simulink library "Powertrain_Library_GenAI"  (R2024a)
settings: Solver=VariableStepAuto  StartTime=0.0  StopTime=10.0  RelTol=1e-3
undefined symbols (not defined in the file or in its folder): DriveCycle
libraries: simulink x8, slpidlib x1
(part 1 of 2)
settings Model: Creator=LENOVO THINKPAD  LastModifiedBy=malikr2
settings RTWCC: GPUComputeCapability=3.5

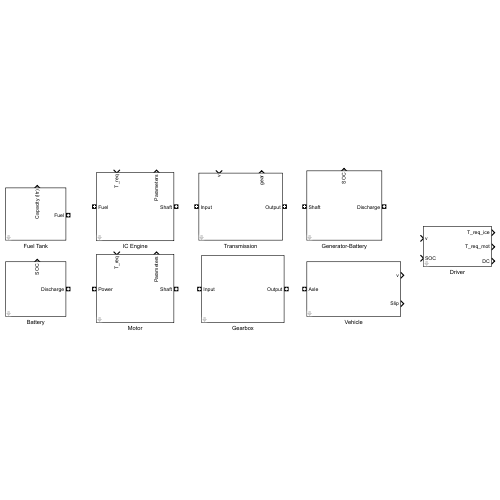
[thumbnail: Simulink's stored preview of the top-level diagram]
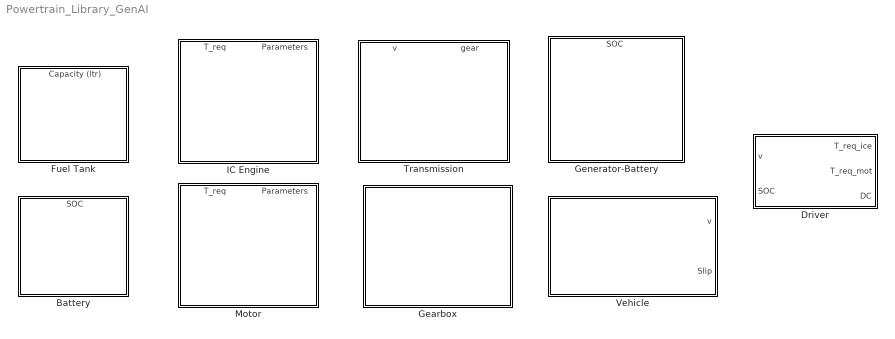
== system Powertrain_Library_GenAI ==
  Battery : Subsystem  mask{V_bat_nom=228, R_bat=0.1037, mAh_bat_rated=87500, SOC_bat_0=1, min_SOC=0.2, attribute_vector={'STORE', 'BAT', '1', {'ELEC'}, {'OUT'}}, cost=4000, base_emissions=8000}
      mask prompts: V_bat_nom "Battery Nominal Voltage (V)"; R_bat "Battery Internal Resistance (Ohm)"; mAh_bat_rated "Battery Capacity (mAh)"; SOC_bat_0 "Initial SOC"; min_SOC "Minimum Operable SOC"; cost "Cost (Euros)"; base_emissions "Production Emissions (kg of CO2)"
      settings: PortSchema="{\"entries\":[{\"content\":{\"sides\":[{\"content\":{},\"type\":\"ConnectorPlacement.EquallySpacedRectSide\",\"uuid\":\"791ecc86-3bcc-4c6a-a153-95c10547b091\"},{\"content\":{\"connectorIds\":[\"RConn1\"],\"side\":\"RIGHT\"},\"type\":\"ConnectorPlacement.EquallySpacedRectSide\",\"uuid\":\"8e54d6b5-5ca6-4d71-8ac9-0532fb867ed6\"},{\"content\":{\"connectorIds\":[\"Out1\"],\"side\":\"TOP\"},\"type\":\"ConnectorPlacement.EquallySpacedRectSide\",\"uuid\":\"933f38fd-4181-4d8b-8acd-50ce6fa4b91a\"}]},\"type\":\"ConnectorPlacement.EquallySpacedConnector\",\"uuid\":\"308b2aba-12b6-4e08-8192-d5b89fa1859a\"}],\"packageUris\":[\"http://schema.mathworks.com/mf0/Connector/R2020b\"],\"version\":\"1.0\"}"
      mask DialogControl Container3 Prompt: Economic Parameters
  Driver : Subsystem  mask{K_p=0, K_i=0, K_d=0, drive_cycle=DriveCycle, ITAE=0, attribute_vector={'CONTROLLER', 'DRV', '0', {}, ''}, series_hybrid_mode=0, charging_torque=50, charging_time=60, min_charge_SOC=0.5}
      mask prompts: K_p "Proportional Gain"; K_i "Integral Gain"; K_d "Derivative Gain"; drive_cycle "Drive Cycle"; series_hybrid_mode "Series Hybrid Mode"; charging_torque "Charging Torque (Nm)"; charging_time "Charging time (seconds)"; min_charge_SOC "Min. SOC to start charging"
      mask DialogControl Container3 Prompt: Hybrid Control
  Fuel Tank : Subsystem  mask{Parameter1=0, attribute_vector={'STORE', 'FT', '1', {'CHEM'}, {'OUT'}}, fuel_energy_density=46, fuel_density=750, fuel_capacity=4, cost=300, base_emissions=200}
      mask prompts: fuel_energy_density "Fuel Energy Density (MJ/kg)"; fuel_density "Fuel Density (kg/m^3)"; fuel_capacity "Tank Capacity (litres)"; cost "Cost (Euros)"; base_emissions "Production Emissions (kg of CO2)"
      settings: PortSchema="{\"entries\":[{\"content\":{\"sides\":[{\"content\":{},\"type\":\"ConnectorPlacement.EquallySpacedRectSide\",\"uuid\":\"791ecc86-3bcc-4c6a-a153-95c10547b091\"},{\"content\":{\"connectorIds\":[\"RConn1\"],\"side\":\"RIGHT\"},\"type\":\"ConnectorPlacement.EquallySpacedRectSide\",\"uuid\":\"8e54d6b5-5ca6-4d71-8ac9-0532fb867ed6\"},{\"content\":{\"connectorIds\":[\"Out1\"],\"side\":\"TOP\"},\"type\":\"ConnectorPlacement.EquallySpacedRectSide\",\"uuid\":\"933f38fd-4181-4d8b-8acd-50ce6fa4b91a\"}]},\"type\":\"ConnectorPlacement.EquallySpacedConnector\",\"uuid\":\"308b2aba-12b6-4e08-8192-d5b89fa1859a\"}],\"packageUris\":[\"http://schema.mathworks.com/mf0/Connector/R2020b\"],\"version\":\"1.0\"}"
      mask DialogControl Container3 Prompt: Economic Parameters
  Gearbox : Subsystem  mask{G=9, eff_gb=0.96, attribute_vector={'TRANSMIT', 'GB', '2', {'MECH', 'MECH'}, {'IN','OUT'}}, cost=1200, base_emissions=1000}
      mask prompts: G "Gear Ratio"; eff_gb "Gearbox Efficiency"; cost "Cost (Euros)"; base_emissions "Production Emissions (kg of CO2)"
      mask DialogControl Container3 Prompt: Economic Parameters
  Generator-Battery : Subsystem  mask{eff_gen=0.85, generator_rpm=6000, V_bat_nom=228, R_bat=0.1037, mAh_bat_rated=87500, SOC_bat_0=0.6, min_SOC=0.2, attribute_vector={'GENERATOR', 'GEN', '2', {'MECH','ELEC'}, {'IN','OUT'}}, cost=7500, base_emissions=10000}
      mask prompts: eff_gen "Generator Efficiency"; generator_rpm "Generator Working Speed (RPM)"; V_bat_nom "Battery Nominal Voltage (V)"; R_bat "Battery Internal Resistance (Ohm)"; mAh_bat_rated "Battery Capacity (mAh)"; SOC_bat_0 "Initial SOC"; min_SOC "Minimum Operable SOC"; cost "Cost (Euros)"; base_emissions "Production Emissions (kg of CO2)"
      settings: PortSchema="{\"entries\":[{\"content\":{\"sides\":[{\"content\":{\"connectorIds\":[\"LConn1\"]},\"type\":\"ConnectorPlacement.EquallySpacedRectSide\",\"uuid\":\"a8b73504-e9cb-44b1-bc91-1a2623164e75\"},{\"content\":{\"connectorIds\":[\"RConn1\"],\"side\":\"RIGHT\"},\"type\":\"ConnectorPlacement.EquallySpacedRectSide\",\"uuid\":\"a3351110-409d-4b78-bb75-8efa6d683458\"},{\"content\":{\"connectorIds\":[\"Out1\"],\"side\":\"TOP\"},\"type\":\"ConnectorPlacement.EquallySpacedRectSide\",\"uuid\":\"2c783bb7-545b-4095-8c4d-b76f612407dc\"}]},\"type\":\"ConnectorPlacement.EquallySpacedConnector\",\"uuid\":\"3e5aa339-5af4-4070-a704-22faf7e6b2c2\"}],\"packageUris\":[\"http://schema.mathworks.com/mf0/Connector/R2020b\"],\"version\":\"1.0\"}"
      mask DialogControl Container4 Prompt: Generator Parameters
      mask DialogControl ParameterGroupVar Prompt: Battery Parameters
      mask DialogControl Container3 Prompt: Economic Parameters
  IC Engine : Subsystem  mask{torque_modelling=Normalized 3rd-order polynomial approximation, efficiency_modelling=Variable Efficiency, attribute_vector={'ACTUATOR', 'ICE', '2', {'CHEM','MECH'}, {'IN','OUT'}}, P_p=125000, T_p=228, w_P=6000, w_T=4500, w_ice_max=7000, w_ice_stall=1000, T_ice_data=[180, 192, 207, 215, 220, 225, 228, 226, 220, 210, 200, 182, 162], w_ice_data=[1000, 1500, 2000, 2500, 3000, 3500, 4000, 4500, 5000, 5500, 6000, 6500, 7000], eff_ice_avg=0.25, eff_ice_data=[0.0900 0.0900 0.0900 0.0900 0.0900 0.0900 0.0850 0.0800 0.0750 0.0700 0.0500;         0.1700 0.1700 0.1700 0.1700 0.1600 0.1500 0.1400 0.1300 0.1200 0.1100 0.0900;         0.2100 0.2100 0.2100 0.2100 0.2100 0.2050 0.2000 0.1800 0.1650 0.1500 0.1300;         0.2500 0.2500 0.2500 0.2500 0.2400 0.2350 0.2200 0.2050 0.1900 0.1700 0.1500;         0.2650 0.2700 0.2700 0.2700 0.2650 0.2500 0.2450 0.2350 0.2150 0.1950 0.1700;         0.2800 0.2800 0.2800 0.2800 0.2800 0.2700 0.2650 0.2500 0.2300 0.2100 0.1900;         0.3000 0.3000 0.3000 0.3000 0.3000 0.3000 0.2900 0.2700 0.2500 0.2150 0.1900;         0.3200 0.3300 0.3300 0.3300 0.3300 0.3300 0.3100 0.2750 0.2400 0.2050 0.1800;         0.2900 0.3100 0.3400 0.3400 0.3300 0.3000 0.2700 0.2500 0.2300 0.1900 0.1700;         0.2500 0.2800 0.3150 0.3150 0.2900 0.2700 0.2500 0.2300 0.2200 0.1800 0.1600;         0.2500 0.2800 0.3150 0.3150 0.2900 0.2700 0.2500 0.2300 0.2200 0.1800 0.1600], T_ice_norm_data=[0; 25; 50; 75; 100; 125; 150; 175; 200; 225; 228]/228, w_ice_norm_data=[1000 1600 2200 2800 3400 4000 4600 5200 5800 6300 7000]/7000, cost=2500, base_emissions=3000}
      mask prompts: torque_modelling "Model Parameterization"; efficiency_modelling "Efficiency Modelling"; P_p "Max. Power (W)"; T_p "Max. Torque (Nm)"; w_P "Speed @ Max. Power (rpm)"; w_T "Speed @ Max. Torque (rpm)"; w_ice_max "Max. Speed (rpm)"; w_ice_stall "Stall Speed (rpm)"; T_ice_data "Torque values (Nm)"; w_ice_data "Speed breakpoints (rpm)"; eff_ice_avg "Average Engine Efficiency"; eff_ice_data "Engine Efficiency map data"; T_ice_norm_data "Torque breakpoints (normalized w.r.t max. torque)"; w_ice_norm_data "Speed breakpoints (normalized w.r.t max. speed)"; cost "Cost (Euros)"; base_emissions "Production Emissions (kg of CO2)"
      settings: PortSchema="{\"entries\":[{\"content\":{\"sides\":[{\"content\":{\"connectorIds\":[\"LConn1\"]},\"type\":\"ConnectorPlacement.EquallySpacedRectSide\",\"uuid\":\"10ac0862-84c0-40da-a453-235e59b4628d\"},{\"content\":{\"connectorIds\":[\"RConn1\"],\"side\":\"RIGHT\"},\"type\":\"ConnectorPlacement.EquallySpacedRectSide\",\"uuid\":\"cd810463-95cc-48e1-84e4-d50e07225fce\"},{\"content\":{\"connectorIds\":[\"In1\",\"Out1\"],\"side\":\"TOP\"},\"type\":\"ConnectorPlacement.EquallySpacedRectSide\",\"uuid\":\"990bc9f6-9b76-43af-8727-286cb1281cc3\"}]},\"type\":\"ConnectorPlacement.EquallySpacedConnector\",\"uuid\":\"ec51f7b2-97ac-4e7c-b90f-37b44cc14701\"}],\"packageUris\":[\"http://schema.mathworks.com/mf0/Connector/R2020b\"],\"version\":\"1.0\"}"
      mask TypeOptions torque_modelling: ICE_Torque_Limits/torque_modelling
      mask TypeOptions efficiency_modelling: ICE_Efficiency/efficiency_modelling
      mask TypeOptions P_p: ICE_Torque_Limits/P_p
      mask TypeOptions T_p: ICE_Torque_Limits/T_p
      mask TypeOptions w_P: ICE_Torque_Limits/w_P
      mask TypeOptions w_T: ICE_Torque_Limits/w_T
      mask TypeOptions w_ice_max: ICE_Torque_Limits/w_ice_max
      mask TypeOptions w_ice_stall: ICE_Torque_Limits/w_ice_stall
      mask TypeOptions T_ice_data: ICE_Torque_Limits/T_ice_data
      mask TypeOptions w_ice_data: ICE_Torque_Limits/w_ice_data
      mask TypeOptions eff_ice_avg: ICE_Efficiency/eff_ice_avg
      mask TypeOptions eff_ice_data: ICE_Efficiency/eff_ice_data
      mask TypeOptions T_ice_norm_data: ICE_Efficiency/T_ice_norm_data
      mask TypeOptions w_ice_norm_data: ICE_Efficiency/w_ice_norm_data
      mask DialogControl Container3 Prompt: Polynomial Approximation Parameters
      mask DialogControl Container4 Prompt: Torque Curve Data
      mask DialogControl Control2 Prompt: Torque Curve
      mask DialogControl Container6 Prompt: Constant Efficiency Modelling
      mask DialogControl Container5 Prompt: Efficiency Map Modelling
      mask DialogControl Container7 Prompt: Economic Parameters
      mask DialogControl Control3 Prompt: Efficiency Map
  Motor : Subsystem  mask{attribute_vector={'ACTUATOR', 'MOT', '2', {'ELEC','MECH'}, {'IN','OUT'}}, mot_efficiency_modelling=Constant Efficiency, T_mot_max=265, P_mot_max=140000, w_mot_max=20000, eff_mot_avg=0.85, eff_mot_data=[0.5833    0.6122    0.7211    0.7696    0.7951    0.8158    0.8293    0.8392    0.8475    0.8519    0.8536    0.8549    0.8563    0.8593    0.8607    0.8605    0.8610    0.8604    0.8590    0.8578    0.8583    0.8582    0.8571    0.8549    0.8535    0.8511    0.8486    0.8479    0.8478    0.8475    0.8431    0.8384    0.8350;     0.5833    0.6122    0.7211    0.7696    0.7951    0.8158    0.8293    0.8392    0.8475    0.8519    0.8536    0.8549    0.8563    0.8593    0.8607    0.8605    0.8610    0.8604    0.8590    0.8578    0.8583    0.8582    0.8571    0.8549    0.8535    0.8511    0.8486    0.8479    0.8478    0.8475    0.8431    0.8384    0.8350;     0.5833    0.6122    0.7211    0.7696    0.7951    0.8158    0.8293    0.8392    0.8475    0.8519    0.8536    0.8549    0.8563    0.8593    0.8607    0.8605    0.8610    0.8604    0.8590    0.8578    0.8583    0.8582    0.8571    0.8549    0.8535    0.8511    0.8486    0.8479    0.8478    0.8475    0.8431    0.8384    0.8350;     0.6173    0.6437    0.7458    0.7900    0.8162    0.8329    0.8454    0.8553    0.8632    0.8680    0.8706    0.8725    0.8742    0.8766    0.8773    0.8778    0.8785    0.8782    0.8771    0.8768    0.8773    0.8779    0.8770    0.8755    0.8745    0.8726    0.8708    0.8700    0.8697    0.8690    0.8650    0.8610    0.8577;     0.6598    0.6830    0.7767    0.8155    0.8427    0.8543    0.8657    0.8756    0.8830    0.8884    0.8921    0.8951    0.8970    0.8988    0.8985    0.8998    0.9009    0.9008    0.9002    0.9010    0.9016    0.9030    0.9024    0.9018    0.9014    0.9003    0.8991    0.8982    0.8976    0.8963    0.8928    0.8897    0.8865;     0.6882    0.7100    0.7974    0.8327    0.8575    0.8677    0.8780    0.8872    0.8944    0.8993    0.9038    0.9070    0.9084    0.9107    0.9106    0.9121    0.9136    0.9008    0.9002    0.9010    0.9016    0.9030    0.9024    0.9018    0.9014    0.9003    0.8991    0.8982    0.8976    0.9114    0.9087    0.9061    0.9036;     0.7106    0.7317    0.8136    0.8462    0.8670    0.8776    0.8866    0.8946    0.9015    0.9054    0.9106    0.9135    0.9138    0.9174    0.9180    0.9194    0.9214    0.9201    0.9233    0.9259    0.9266    0.9270    0.9265    0.9258    0.9255    0.9246    0.9231    0.9220    0.9209    0.9199    0.9182    0.9158    0.9145;     0.7300    0.7502    0.8257    0.8561    0.8740    0.8841    0.8931    0.9005    0.9069    0.9106    0.9162    0.9189    0.9191    0.9228    0.9240    0.9251    0.9274    0.9261    0.9301    0.9329    0.9337    0.9335    0.9329    0.9319    0.9316    0.9305    0.9292    0.9284    0.9275    0.9268    0.9259    0.9231    0.9222;     0.7462    0.7649    0.8331    0.8620    0.8782    0.8868    0.8974    0.9048    0.9103    0.9148    0.9205    0.9231    0.9243    0.9265    0.9284    0.9291    0.9314    0.9311    0.9344    0.9365    0.9375    0.9369    0.9362    0.9350    0.9346    0.9333    0.9328    0.9325    0.9323    0.9320    0.9316    0.9276    0.9265;     0.7603    0.7775    0.8395    0.8665    0.8811    0.8889    0.9006    0.9079    0.9130    0.9180    0.9238    0.9263    0.9281    0.9296    0.9318    0.9323    0.9345    0.9351    0.9378    0.9393    0.9404    0.9395    0.9388    0.9377    0.9373    0.9358    0.9362    0.9363    0.9366    0.9364    0.9365    0.9325    0.9312;     0.7688    0.7847    0.8434    0.8680    0.8812    0.8896    0.9009    0.9082    0.9144    0.9191    0.9246    0.9275    0.9289    0.9308    0.9326    0.9335    0.9352    0.9367    0.9392    0.9402    0.9412    0.9404    0.9397    0.9394    0.9394    0.9374    0.9393    0.9393    0.9399    0.9390    0.9390    0.9384    0.9369;     0.7770    0.7917    0.8473    0.8696    0.8815    0.8905    0.9013    0.9087    0.9157    0.9202    0.9255    0.9287    0.9299    0.9322    0.9337    0.9351    0.9363    0.9386    0.9409    0.9414    0.9423    0.9416    0.9410    0.9414    0.9416    0.9392    0.9423    0.9422    0.9431    0.9418    0.9414    0.9392    0.9366;     0.7816 ...(+9613 chars)], T_mot_norm_data=[0    0.0250    0.0500    0.0750    0.1000    0.1250    0.1500    0.1750    0.2000    0.2250    0.2500    0.2750    0.3000    0.3250    0.3500    0.3750    0.4000    0.4250    0.4500    0.4750    0.5000    0.5250    0.5500    0.5750    0.6000    0.6250    0.6500    0.6750    0.7000    0.7250    0.7500    0.7750    0.8000    0.8250    0.8500    0.8750    0.9000    0.9250    0.9500    0.9750    1.0000], w_mot_norm_data=[0    0.0312    0.0625    0.0938    0.1250    0.1562    0.1875    0.2188    0.2500    0.2812    0.3125    0.3438    0.3750    0.4062    0.4375    0.4688    0.5000    0.5313    0.5625    0.5938    0.6250    0.6563    0.6875    0.7188    0.7500    0.7813    0.8125    0.8438    0.8750    0.9063    0.9375    0.9688    1.0000], cost=3500, base_emissions=2000}
      mask prompts: mot_efficiency_modelling "Efficiency Modelling"; T_mot_max "Max. Torque (Nm)"; P_mot_max "Max. Power (W)"; w_mot_max "Max. Speed (rpm)"; eff_mot_avg "Average Motor Efficiency"; eff_mot_data "Motor Efficiency map data"; T_mot_norm_data "Torque breakpoints (normalized w.r.t max. torque)"; w_mot_norm_data "Speed breakpoints (normalized w.r.t max. speed)"; cost "Cost (Euros)"; base_emissions "Production Emissions (kg of CO2)"
      mask init:
      | choice = get_param(gcb,'mot_efficiency_modelling');
      | vssBlk = gcb;
      | oldVariant = get_param(gcb,'LabelModeActiveChoice');
      | if strcmp(choice,'Constant Efficiency')
      |     
      |     set_param(vssBlk, 'LabelModeActiveChoice', 'Constant Efficiency');
      | else
      |     
      |     set_param(vssBlk, 'LabelModeActiveChoice', 'Variable Efficiency');
      | end
      settings: PortSchema="{\"entries\":[{\"content\":{\"sides\":[{\"content\":{\"connectorIds\":[\"LConn1\"]},\"type\":\"ConnectorPlacement.EquallySpacedRectSide\",\"uuid\":\"d69cc2a8-6a3c-4a8d-b68e-91d71b395a3b\"},{\"content\":{\"connectorIds\":[\"RConn1\"],\"side\":\"RIGHT\"},\"type\":\"ConnectorPlacement.EquallySpacedRectSide\",\"uuid\":\"d647e5ef-109d-4ce3-ab7e-e6a182f65a21\"},{\"content\":{\"connectorIds\":[\"In1\",\"Out1\"],\"side\":\"TOP\"},\"type\":\"ConnectorPlacement.EquallySpacedRectSide\",\"uuid\":\"312f8dd1-64ed-4775-9005-2e4b9713465a\"}]},\"type\":\"ConnectorPlacement.EquallySpacedConnector\",\"uuid\":\"f649af3d-7f9c-439b-b818-7c0a660138bb\"}],\"packageUris\":[\"http://schema.mathworks.com/mf0/Connector/R2020b\"],\"version\":\"1.0\"}"
      mask TypeOptions mot_efficiency_modelling: Constant Efficiency | Variable Efficiency
      mask DialogControl Container3 Prompt: Constant Efficiency Modelling
      mask DialogControl Container4 Prompt: Efficiency Map Modelling
      mask DialogControl Container5 Prompt: Economic Parameters
  Transmission : Subsystem  mask{Gs=[3.07 1.77 1.19 0.87 0.7], shift_thresholds=[10 30 50 75], eff_tr=0.95, attribute_vector={'TRANSMIT', 'TR', '2', {'MECH', 'MECH'}, {'IN','OUT'}}, cost=2000, base_emissions=1500}
      mask prompts: Gs "Gear Ratios"; shift_thresholds "Shifting Speeds"; eff_tr "Transmission Efficiency"; cost "Cost (Euros)"; base_emissions "Production Emissions (kg of CO2)"
      settings: PortSchema="{\"entries\":[{\"content\":{\"sides\":[{\"content\":{\"connectorIds\":[\"LConn1\"]},\"type\":\"ConnectorPlacement.EquallySpacedRectSide\",\"uuid\":\"d09a0a32-443c-4f9e-91dd-87ec36bd85ce\"},{\"content\":{\"connectorIds\":[\"RConn1\"],\"side\":\"RIGHT\"},\"type\":\"ConnectorPlacement.EquallySpacedRectSide\",\"uuid\":\"d259d690-b55a-4cd8-8e7c-4fe36dc86a09\"},{\"content\":{\"connectorIds\":[\"In1\",\"Out1\"],\"side\":\"TOP\"},\"type\":\"ConnectorPlacement.EquallySpacedRectSide\",\"uuid\":\"57e7772c-c7c4-45ad-8d76-bdaa2e04622c\"}]},\"type\":\"ConnectorPlacement.EquallySpacedConnector\",\"uuid\":\"0ab49f07-500b-4369-8c08-c0971259b237\"}],\"packageUris\":[\"http://schema.mathworks.com/mf0/Connector/R2020b\"],\"version\":\"1.0\"}"
      mask DialogControl Container3 Prompt: Economic Parameters
  Vehicle : Subsystem  mask{m=1800, r=0.335, A=2.2, C_D=0.23, mu_rr=0.008, mu_fr=0.7, rho=1.13, g=9.81, attribute_vector={'LOAD', 'VEH', '1', {'MECH'}, {'IN'}}, cost=1500, base_emissions=1500}
      mask prompts: m "Mass (kg)"; r "Tire Radius (m)"; A "Frontal Area (m^2)"; C_D "Drag Coefficient"; mu_rr "Rolling Resistance Coefficient"; mu_fr "Road Friction Coefficient"; rho "Air Density (kg/m^3)"; g "Acceleration due to gravity (m/s^2)"; cost "Cost (Euros)"; base_emissions "Production Emissions (kg of CO2)"
      mask DialogControl Container3 Prompt: Economic Parameters

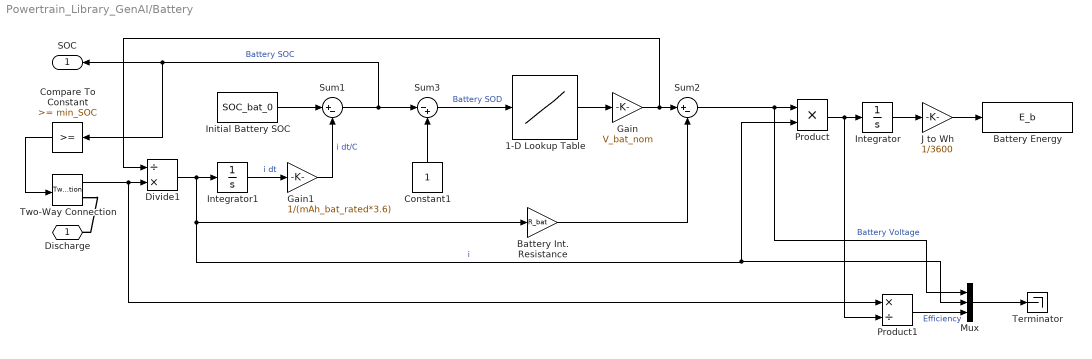
== system Powertrain_Library_GenAI/Battery ==
  1-D Lookup Table : Lookup_n-D  NumberOfTableDimensions=1  BreakpointsForDimension1=[0 0.0278 0.0722 0.1111 0.1500 0.2028 0.2694 0.3389 0.4139 0.4917 0.5528 0.6111 0.6639 0.7306 0.8111 0.8806 1.0000 1.0861 1.1861 1.2889 1.3917 1.4778 1.5722 1.6556 1.7444 1.8306 1.9194 2.0083 2.1056 2.1778 2.2917 2.4000 2.5111 2.6194 2.7333 2.8167 2.8889 2.9500 3.0028 3.0556 3.1083 3.1583 3.2111 3.2444 3.2694 3.2861]/3.2861  Table=[4.0700 3.9545 3.9221 3.9026 3.8896 3.8669 3.8474 3.8279 3.7987 3.7727 3.7468 3.7305 3.7110 3.6916 3.6688 3.6461 3.6136 3.5877 3.5552 3.5227 3.4903 3.4643 3.4383 3.4156 3.3929 3.3734 3.3539 3.3312 3.3149 3.2987 3.2662 3.2403 3.2078 3.1688 3.1266 3.0909 3.0519 3.0162 2.9773 2.9351 2.8799 2.8084 2.7175 2.6461 2.5682 2.4968]/4.0700  InternalRulePriority=Speed  RndMeth=Simplest
  Battery Energy : ToWorkspace  VariableName=E_b  SaveFormat=Timeseries  SampleTime=-1
  Battery Int. Resistance : Gain  Gain=R_bat
  Compare To Constant : simulink/Logic and Bit Operations/Compare To Constant  relop=>=  const=min_SOC  OutDataTypeStr=uint8  ZeroCross=off
  Constant1 : Constant
  Divide1 : Product  Inputs=/*
  Gain : Gain  Gain=V_bat_nom
  Gain1 : Gain  Gain=1/(mAh_bat_rated*3.6)
  Initial Battery SOC : Constant  Value=SOC_bat_0
  Integrator : Integrator  ZeroCross=off
  Integrator1 : Integrator
  J to Wh : Gain  Gain=1/3600
  Mux : Mux  Inputs=3
  Product : Product
  Product1 : Product  Inputs=*/
  Sum1 : Sum  Inputs=|+-
  Sum2 : Sum  Inputs=|+-
  Sum3 : Sum  Inputs=|-+
  Terminator : Terminator
  Two-Way Connection : TwoWayConnection
  Discharge : PMIOPort  Side=Right
  SOC : Outport
  wires:
  Integrator/1 -> J to Wh/1
  J to Wh/1 -> Battery Energy/1
  Compare To Constant/1 -> Two-Way Connection/1
  Initial Battery SOC/1 -> Sum1/1
  Sum2/1 -> Mux/1, Product/1  "Battery Voltage"
  Product/1 -> Product1/2, Integrator/1
  Integrator1/1 -> Gain1/1  "i dt"
  Battery Int. Resistance/1 -> Sum2/2
  Gain1/1 -> Sum1/2  "i dt/C"
  Two-Way Connection/1 -> Product1/1, Divide1/2
  Sum3/1 -> 1-D Lookup Table/1  "Battery SOD"
  Divide1/1 -> Integrator1/1, Battery Int. Resistance/1, Mux/2, Product/2  "i"
  Sum1/1 -> Sum3/1, Compare To Constant/1, SOC/1  "Battery SOC"
  Constant1/1 -> Sum3/2
  Mux/1 -> Terminator/1
  Product1/1 -> Mux/3  "Efficiency"
  Gain/1 -> Divide1/1, Sum2/1
  1-D Lookup Table/1 -> Gain/1
  connections:
  Two-Way Connection/RConn1 -- Discharge/RConn1

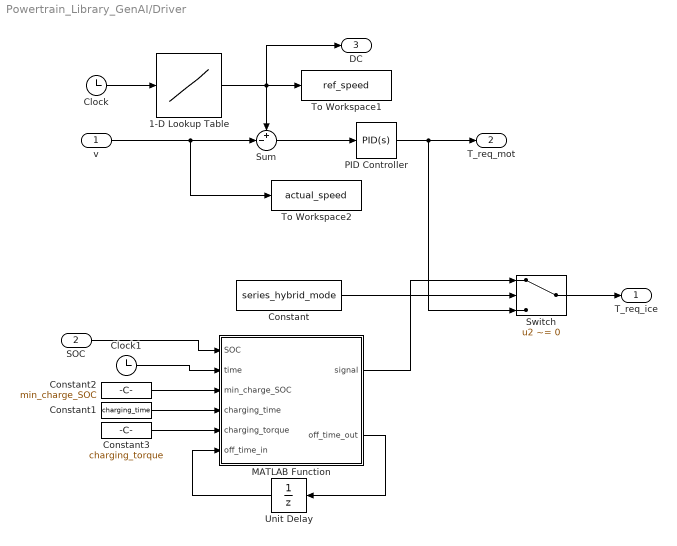
== system Powertrain_Library_GenAI/Driver ==
  v : Inport
  SOC : Inport  Port=2
  1-D Lookup Table : Lookup_n-D  NumberOfTableDimensions=1  BreakpointsForDimension1=drive_cycle(:,1)  Table=drive_cycle(:,2)  InternalRulePriority=Speed  RndMeth=Simplest
  Clock : Clock
  Clock1 : Clock
  Constant : Constant  Value=series_hybrid_mode
  Constant1 : Constant  Value=charging_time
  Constant2 : Constant  Value=min_charge_SOC
  Constant3 : Constant  Value=charging_torque
  MATLAB Function : MATLAB Function  TreatAsAtomicUnit=on
  PID Controller : slpidlib/PID Controller  Controller=PID  Form=Parallel  TimeDomain=Continuous-time  UseExternalTs=off  SampleTime=-1  IntegratorMethod=Forward Euler  FilterMethod=Forward Euler  ControllerParametersSource=internal  P=K_p  I=K_i  UseKiTs=off  D=K_d  UseExternalDerivativeSource=off  N=100  UseFilter=on  TunerSelectOption=Transfer Function Based (PID Tuner App)  InitialConditionSource=internal  InitialConditionForIntegrator=0  InitialConditionForFilter=0  DifferentiatorICPrevScaledInput=0  ExternalReset=none  TrackingMode=off  Kt=1  LimitOutput=off  SatLimitsSource=internal  UpperSaturationLimit=inf  LowerSaturationLimit=-inf  LinearizeAsGain=on  AntiWindupMode=none  Kb=1  LimitIntegrator=off  UpperIntegratorSaturationLimit=inf  LowerIntegratorSaturationLimit=-inf  POutMin=[]  POutMax=[]  IOutMin=[]  IOutMax=[]  DOutMin=[]  DOutMax=[]  NOutMin=[]  NOutMax=[]  SumOutMin=[]  SumOutMax=[]  SaturationOutMin=[]  SaturationOutMax=[]  PParamMin=[]  PParamMax=[]  IParamMin=[]  IParamMax=[]  DParamMin=[]  DParamMax=[]  NParamMin=[]  NParamMax=[]  KbParamMin=[]  KbParamMax=[]  KtParamMin=[]  KtParamMax=[]  KbOutMin=[]  KbOutMax=[]  KtOutMin=[]  KtOutMax=[]  IntegratorOutMin=[]  IntegratorOutMax=[]  FilterOutMin=[]  FilterOutMax=[]  SumI1OutMin=[]  SumI1OutMax=[]  SumI2OutMin=[]  SumI2OutMax=[]  SumI3OutMin=[]  SumI3OutMax=[]  SumI4OutMin=[]  SumI4OutMax=[]  SumDOutMin=[]  SumDOutMax=[]  DifferentiatorOutMin=[]  DifferentiatorOutMax=[]  FilterDiffOutCoefMin=[]  FilterDiffOutCoefMax=[]  ReciprocalOutMin=[]  ReciprocalOutMax=[]  SumDenOutMin=[]  SumDenOutMax=[]  SumNumOutMin=[]  SumNumOutMax=[]  DivideOutMin=[]  DivideOutMax=[]  UdiffTsProdOutMin=[]  UdiffTsProdOutMax=[]  NTsProdOutMin=[]  NTsProdOutMax=[]  UintegralTsProdOutMin=[]  UintegralTsProdOutMax=[]  UngainTsProdOutMin=[]  UngainTsProdOutMax=[]  ClampingZeroOutDataTypeStr=Inherit: Inherit via back propagation  ClampingZeroOutMin=[]  ClampingZeroOutMax=[]  FilterDenConstantOutDataTypeStr=Inherit: Inherit via back propagation  FilterDenConstantOutMin=[]  FilterDenConstantOutMax=[]  PCopyOutDataTypeStr=Inherit: Inherit via back propagation  PCopyOutMin=[]  PCopyOutMax=[]  NCopyOutDataTypeStr=Inherit: Inherit via back propagation  NCopyOutMin=[]  NCopyOutMax=[]  IntegratorContinuousStateAttributes=''  IntegratorStateMustResolveToSignalObject=off  IntegratorRTWStateStorageClass=Auto  FilterContinuousStateAttributes=''  FilterStateMustResolveToSignalObject=off  FilterRTWStateStorageClass=Auto  ParallelPVariant=InternalParameters  IdealPVariant=Disabled  IVariant=InternalParameters  DVariant=InternalParameters  IntegratorVariant=Continuous  SatVariant=Disabled  AWVariant=Passthrough  PCopyVariant=Disabled  TRVariant=Disabled  FdbkBlocksVariant=Forward  IdealPFdbkVariant=Disabled  SatFdbkVariant=Disabled  DerivativeFilterVariant=ContFilter  NVariant=InternalParameters  NCopyVariant=Disabled  FilterICVariant=InternalICsFilter  IntegratorICVariant=InternalICs  ExternalResetVariant=Disabled  TRSumVariant=Passthrough  SumFdbkVariant=Disabled  SumVariant=Sum_PID  TsampFilterVariant=InternalTs  TsampNgainVariant=Passthrough  TsampIntegralVariant=Disabled_SignalSpec  ExternalSaturationOutDataTypeStr=Inherit: Same as second input  DerivativeSourceVariant=ErrorSignal
  Sum : Sum  Inputs=+-|
  Switch : Switch  Criteria=u2 ~= 0  SaturateOnIntegerOverflow=off  InputSameDT=off
  To Workspace1 : ToWorkspace  VariableName=ref_speed  SaveFormat=Timeseries  SampleTime=-1
  To Workspace2 : ToWorkspace  VariableName=actual_speed  SaveFormat=Timeseries  SampleTime=-1
  Unit Delay : UnitDelay  SampleTime=-1  HasFrameUpgradeWarning=on
  T_req_ice : Outport
  T_req_mot : Outport  Port=2
  DC : Outport  Port=3
  wires:
  v/1 -> To Workspace2/1, Sum/2
  PID Controller/1 -> Switch/3, T_req_mot/1
  1-D Lookup Table/1 -> DC/1, To Workspace1/1, Sum/1
  Clock/1 -> 1-D Lookup Table/1
  Sum/1 -> PID Controller/1
  Constant/1 -> Switch/2
  MATLAB Function/1(signal) -> Switch/1
  MATLAB Function/2(off_time_out) -> Unit Delay/1
  Constant1/1 -> MATLAB Function/4(charging_time)
  Constant2/1 -> MATLAB Function/3(min_charge_SOC)
  Clock1/1 -> MATLAB Function/2(time)
  SOC/1 -> MATLAB Function/1(SOC)
  Switch/1 -> T_req_ice/1
  Constant3/1 -> MATLAB Function/5(charging_torque)
  Unit Delay/1 -> MATLAB Function/6(off_time_in)

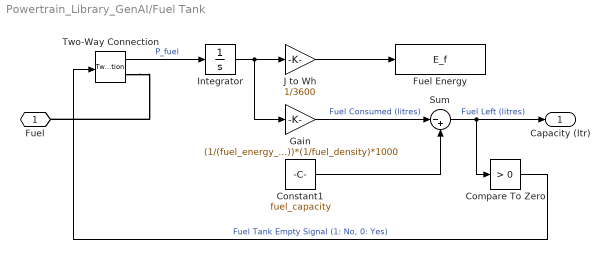
== system Powertrain_Library_GenAI/Fuel Tank ==
  Compare To Zero : simulink/Logic and Bit Operations/Compare To Zero  relop=>  OutDataTypeStr=uint8  ZeroCross=off
  Constant1 : Constant  Value=fuel_capacity
  Fuel Energy : ToWorkspace  VariableName=E_f  SaveFormat=Timeseries  SampleTime=-1
  Gain : Gain  Gain=(1/(fuel_energy_density*10^6))*(1/fuel_density)*1000
  Integrator : Integrator  ZeroCross=off
  J to Wh : Gain  Gain=1/3600
  Sum : Sum  Inputs=|-+
  Two-Way Connection : TwoWayConnection
  Fuel : PMIOPort  Side=Right
  Capacity (ltr) : Outport
  wires:
  Integrator/1 -> Gain/1, J to Wh/1
  Compare To Zero/1 -> Two-Way Connection/1  "Fuel Tank Empty Signal (1: No, 0: Yes)"
  Two-Way Connection/1 -> Integrator/1  "P_fuel"
  J to Wh/1 -> Fuel Energy/1
  Gain/1 -> Sum/1  "Fuel Consumed (litres)"
  Constant1/1 -> Sum/2
  Sum/1 -> Compare To Zero/1, Capacity (ltr)/1  "Fuel Left (litres)"
  connections:
  Two-Way Connection/RConn1 -- Fuel/RConn1

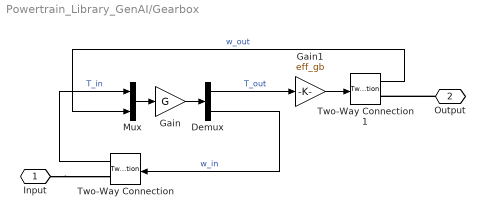
== system Powertrain_Library_GenAI/Gearbox ==
  Demux : Demux  Outputs=2
  Gain : Gain  Gain=G
  Gain1 : Gain  Gain=eff_gb
  Mux : Mux  Inputs=2
  Two-Way Connection : TwoWayConnection
  Two-Way Connection1 : TwoWayConnection
  Input : PMIOPort  Side=Left
  Output : PMIOPort  Port=2  Side=Right
  wires:
  Two-Way Connection/1 -> Mux/1  "T_in"
  Demux/1 -> Gain1/1  "T_out"
  Demux/2 -> Two-Way Connection/1  "w_in"
  Two-Way Connection1/1 -> Mux/2  "w_out"
  Mux/1 -> Gain/1
  Gain/1 -> Demux/1
  Gain1/1 -> Two-Way Connection1/1
  connections:
  Input/RConn1 -- Two-Way Connection/RConn1
  Output/RConn1 -- Two-Way Connection1/RConn1

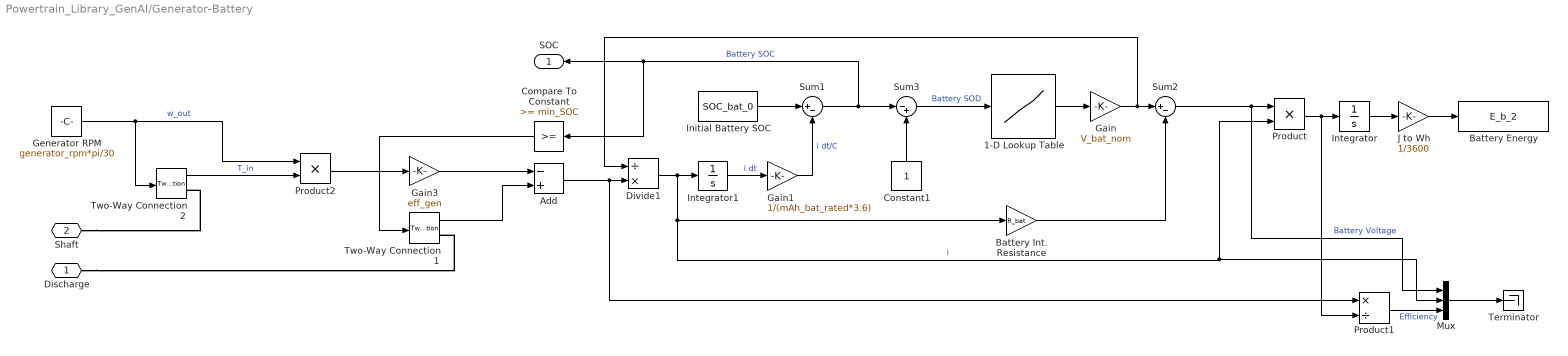
== system Powertrain_Library_GenAI/Generator-Battery ==
  1-D Lookup Table : Lookup_n-D  NumberOfTableDimensions=1  BreakpointsForDimension1=[0 0.0278 0.0722 0.1111 0.1500 0.2028 0.2694 0.3389 0.4139 0.4917 0.5528 0.6111 0.6639 0.7306 0.8111 0.8806 1.0000 1.0861 1.1861 1.2889 1.3917 1.4778 1.5722 1.6556 1.7444 1.8306 1.9194 2.0083 2.1056 2.1778 2.2917 2.4000 2.5111 2.6194 2.7333 2.8167 2.8889 2.9500 3.0028 3.0556 3.1083 3.1583 3.2111 3.2444 3.2694 3.2861]/3.2861  Table=[4.0700 3.9545 3.9221 3.9026 3.8896 3.8669 3.8474 3.8279 3.7987 3.7727 3.7468 3.7305 3.7110 3.6916 3.6688 3.6461 3.6136 3.5877 3.5552 3.5227 3.4903 3.4643 3.4383 3.4156 3.3929 3.3734 3.3539 3.3312 3.3149 3.2987 3.2662 3.2403 3.2078 3.1688 3.1266 3.0909 3.0519 3.0162 2.9773 2.9351 2.8799 2.8084 2.7175 2.6461 2.5682 2.4968]/4.0700  InternalRulePriority=Speed  RndMeth=Simplest
  Add : Sum  Inputs=-+
  Battery Energy : ToWorkspace  VariableName=E_b_2  SaveFormat=Timeseries  SampleTime=-1
  Battery Int. Resistance : Gain  Gain=R_bat
  Compare To Constant : simulink/Logic and Bit Operations/Compare To Constant  relop=>=  const=min_SOC  OutDataTypeStr=uint8  ZeroCross=off
  Constant1 : Constant
  Divide1 : Product  Inputs=/*
  Gain : Gain  Gain=V_bat_nom
  Gain1 : Gain  Gain=1/(mAh_bat_rated*3.6)
  Gain3 : Gain  Gain=eff_gen
  Generator RPM : Constant  Value=generator_rpm*pi/30
  Initial Battery SOC : Constant  Value=SOC_bat_0
  Integrator : Integrator  ZeroCross=off
  Integrator1 : Integrator
  J to Wh : Gain  Gain=1/3600
  Mux : Mux  Inputs=3
  Product : Product
  Product1 : Product  Inputs=*/
  Product2 : Product
  Sum1 : Sum  Inputs=|+-
  Sum2 : Sum  Inputs=|+-
  Sum3 : Sum  Inputs=|-+
  Terminator : Terminator
  Two-Way Connection1 : TwoWayConnection
  Two-Way Connection2 : TwoWayConnection
  Discharge : PMIOPort  Side=Right
  Shaft : PMIOPort  Port=2  Side=Left
  SOC : Outport
  wires:
  Integrator/1 -> J to Wh/1
  J to Wh/1 -> Battery Energy/1
  Compare To Constant/1 -> Two-Way Connection1/1
  Initial Battery SOC/1 -> Sum1/1
  Sum2/1 -> Mux/1, Product/1  "Battery Voltage"
  Product/1 -> Product1/2, Integrator/1
  Integrator1/1 -> Gain1/1  "i dt"
  Battery Int. Resistance/1 -> Sum2/2
  Gain1/1 -> Sum1/2  "i dt/C"
  Add/1 -> Product1/1, Divide1/2
  Sum3/1 -> 1-D Lookup Table/1  "Battery SOD"
  Divide1/1 -> Integrator1/1, Battery Int. Resistance/1, Mux/2, Product/2  "i"
  Sum1/1 -> Sum3/1, Compare To Constant/1, SOC/1  "Battery SOC"
  Constant1/1 -> Sum3/2
  Mux/1 -> Terminator/1
  Product1/1 -> Mux/3  "Efficiency"
  Gain/1 -> Divide1/1, Sum2/1
  1-D Lookup Table/1 -> Gain/1
  Gain3/1 -> Add/1
  Two-Way Connection1/1 -> Add/2
  Generator RPM/1 -> Product2/1, Two-Way Connection2/1  "w_out"
  Two-Way Connection2/1 -> Product2/2  "T_in"
  Product2/1 -> Gain3/1
  connections:
  Discharge/RConn1 -- Two-Way Connection1/RConn1
  Shaft/RConn1 -- Two-Way Connection2/RConn1

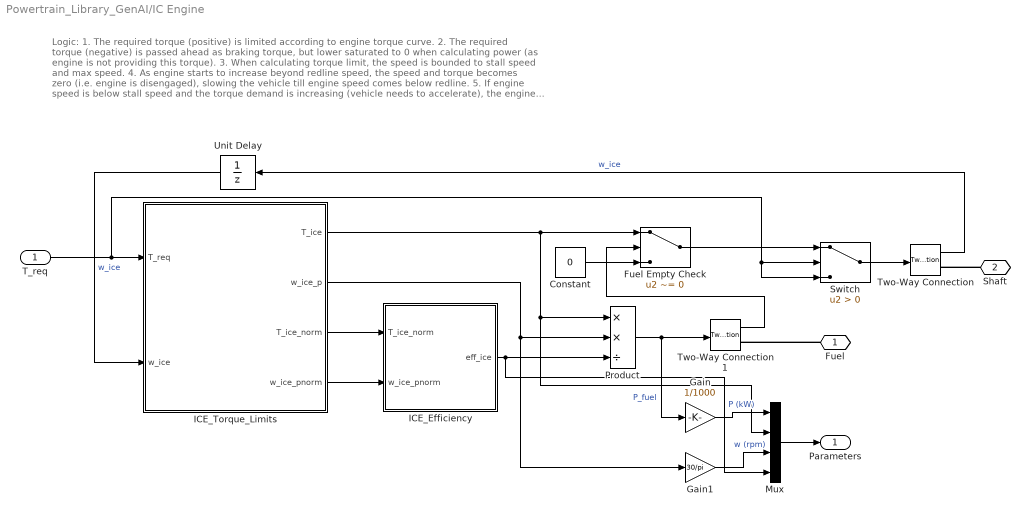
== system Powertrain_Library_GenAI/IC Engine ==
  note: Logic:
      | 1. The required torque (positive) is limited according to engine torque curve.
      | 2. The required torque (negative) is passed ahead as braking torque, but lower saturated to 0 when calculating power (as engine is not providing this torque).
      | 3. When calculating torque limit, the speed is bounded to stall speed and max speed.
      | 4. As engine starts to increase beyond redline speed, the speed and torque becomes zero (i.e. engine is disengaged), slowing the vehicle till engine speed comes below redline.
      | 5. If engine speed is below stall speed and the torque demand is increasing (vehicle needs to accelerate), the engine speed is saturated at stall speed so that it generates torque and thus increases its speed. If torque demand is decreasing (vehicle is decelerating), engine is disengaged so that it stays at stall speed but vehicle does not decrease its speed further.
  T_req : Inport
  Constant : Constant  Value=0
  Fuel Empty Check : Switch  Criteria=u2 ~= 0  SaturateOnIntegerOverflow=off  InputSameDT=off
  Gain : Gain  Gain=1/1000
  Gain1 : Gain  Gain=30/pi
  ICE_Efficiency : Subsystem  Variant=on  VariantControlMode=label  LabelModeActiveChoice=Variable Efficiency  mask{efficiency_modelling=Variable Efficiency, eff_ice_avg=eff_ice_avg, eff_ice_data=eff_ice_data, T_ice_norm_data=T_ice_norm_data, w_ice_norm_data=w_ice_norm_data}
      mask prompts: efficiency_modelling "Efficiency Modelling"
      mask init:
      | choice = get_param(gcb,'efficiency_modelling');
      | vssBlk = gcb;
      | oldVariant = get_param(gcb,'LabelModeActiveChoice');
      | if strcmp(choice,'Constant Efficiency')
      |     
      |     set_param(vssBlk, 'LabelModeActiveChoice', 'Constant Efficiency');
      | else
      |     
      |     set_param(vssBlk, 'LabelModeActiveChoice', 'Variable Efficiency');
      | end
      mask TypeOptions efficiency_modelling: Constant Efficiency | Variable Efficiency
  ICE_Torque_Limits : Subsystem  Variant=on  VariantControlMode=label  LabelModeActiveChoice=Normalized 3rd-order polynomial approximation  mask{torque_modelling=Normalized 3rd-order polynomial approximation, P_p=P_p, T_p=T_p, w_P=w_P, w_T=w_T, w_ice_max=w_ice_max, w_ice_stall=w_ice_stall, w_ice_data=w_ice_data, T_ice_data=T_ice_data}
      mask init:
      | choice = get_param(gcb,'torque_modelling');
      | vssBlk = gcb;
      | oldVariant = get_param(gcb,'LabelModeActiveChoice');
      | if strcmp(choice,'Normalized 3rd-order polynomial approximation')
      |     
      |     set_param(vssBlk, 'LabelModeActiveChoice', 'Normalized 3rd-order polynomial approximation');
      | else
      |     
      |     set_param(vssBlk, 'LabelModeActiveChoice', 'Torque-Speed curve data');
      | end
      mask TypeOptions torque_modelling: Normalized 3rd-order polynomial approximation | Torque-Speed curve data
  Mux : Mux
  Product : Product  Inputs=**/
  Switch : Switch  Criteria=u2 > Threshold  ZeroCross=off  SaturateOnIntegerOverflow=off  InputSameDT=off
  Two-Way Connection : TwoWayConnection
  Two-Way Connection1 : TwoWayConnection
  Unit Delay : UnitDelay  SampleTime=-1  HasFrameUpgradeWarning=on
  Fuel : PMIOPort  Side=Left
  Shaft : PMIOPort  Port=2  Side=Right
  Parameters : Outport
  wires:
  T_req/1 -> Switch/2, Switch/3, ICE_Torque_Limits/1(T_req)
  Gain/1 -> Mux/1  "P (kW)"
  Mux/1 -> Parameters/1
  Gain1/1 -> Mux/3  "w (rpm)"
  Two-Way Connection/1 -> Unit Delay/1  "w_ice"
  ICE_Torque_Limits/1(T_ice) -> Fuel Empty Check/1, Product/1, Mux/2
  Product/1 -> Gain/1, Two-Way Connection1/1  "P_fuel"
  Unit Delay/1 -> ICE_Torque_Limits/2(w_ice)  "w_ice"
  ICE_Torque_Limits/4(w_ice_pnorm) -> ICE_Efficiency/2(w_ice_pnorm)
  ICE_Torque_Limits/3(T_ice_norm) -> ICE_Efficiency/1(T_ice_norm)
  ICE_Efficiency/1(eff_ice) -> Mux/4, Product/3
  ICE_Torque_Limits/2(w_ice_p) -> Product/2, Gain1/1
  Switch/1 -> Two-Way Connection/1
  Two-Way Connection1/1 -> Fuel Empty Check/2
  Constant/1 -> Fuel Empty Check/3
  Fuel Empty Check/1 -> Switch/1
  connections:
  Shaft/RConn1 -- Two-Way Connection/RConn1
  Fuel/RConn1 -- Two-Way Connection1/RConn1

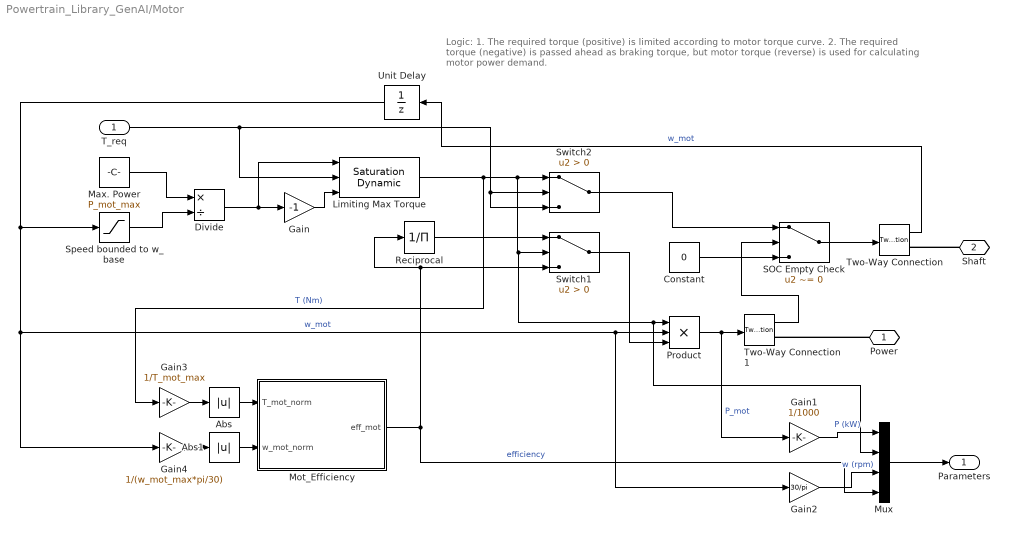
== system Powertrain_Library_GenAI/Motor ==
  note: Logic:
      | 1. The required torque (positive) is limited according to motor torque curve.
      | 2. The required torque (negative) is passed ahead as braking torque, but motor torque (reverse) is used for calculating motor power demand.
  T_req : Inport
  Abs : Abs  SaturateOnIntegerOverflow=off
  Abs1 : Abs  SaturateOnIntegerOverflow=off
  Constant : Constant  Value=0
  Divide : Product  Inputs=*/
  Gain : Gain  Gain=-1
  Gain1 : Gain  Gain=1/1000
  Gain2 : Gain  Gain=30/pi
  Gain3 : Gain  Gain=1/T_mot_max
  Gain4 : Gain  Gain=1/(w_mot_max*pi/30)
  Limiting Max Torque : simulink/Discontinuities/Saturation Dynamic  OutMin=[]  OutMax=[]  OutDataTypeStr=Inherit: Same as second input  OutDataType=fixdt(1, 16)  OutScaling=2^-10  DoSatur=off
  Max. Power : Constant  Value=P_mot_max
  Mot_Efficiency : Subsystem  Variant=on  VariantControlMode=label  LabelModeActiveChoice=Constant Efficiency  mask{mot_efficiency_modelling=Constant Efficiency, eff_mot_avg=eff_mot_avg, eff_mot_data=eff_mot_data, T_mot_norm_data=T_mot_norm_data, w_mot_norm_data=w_mot_norm_data}
      mask TypeOptions mot_efficiency_modelling: Constant Efficiency | Variable Efficiency
  Mux : Mux
  Product : Product  Inputs=3
  Reciprocal : Product  Inputs=/
  SOC Empty Check : Switch  Criteria=u2 ~= 0  SaturateOnIntegerOverflow=off  InputSameDT=off
  Speed bounded to w_base : Saturate  UpperLimit=w_mot_max*pi/30  LowerLimit=P_mot_max/T_mot_max
  Switch1 : Switch  Criteria=u2 > Threshold  SaturateOnIntegerOverflow=off  InputSameDT=off
  Switch2 : Switch  Criteria=u2 > Threshold  SaturateOnIntegerOverflow=off  InputSameDT=off
  Two-Way Connection : TwoWayConnection
  Two-Way Connection1 : TwoWayConnection
  Unit Delay : UnitDelay  SampleTime=-1  HasFrameUpgradeWarning=on
  Power : PMIOPort  Side=Left
  Shaft : PMIOPort  Port=2  Side=Right
  Parameters : Outport
  wires:
  Two-Way Connection/1 -> Unit Delay/1  "w_mot"
  Divide/1 -> Gain/1, Limiting Max Torque/1
  Gain/1 -> Limiting Max Torque/3
  Mot_Efficiency/1(eff_mot) -> Switch1/3, Reciprocal/1, Mux/4  "efficiency"
  Switch1/1 -> Product/3
  Two-Way Connection1/1 -> SOC Empty Check/2
  Max. Power/1 -> Divide/1
  Speed bounded to w_base/1 -> Divide/2
  Product/1 -> Gain1/1, Two-Way Connection1/1  "P_mot"
  T_req/1 -> Limiting Max Torque/2, Switch2/3, Switch2/2
  Unit Delay/1 -> Gain4/1, Gain2/1, Product/2, Speed bounded to w_base/1  "w_mot"
  Gain2/1 -> Mux/3  "w (rpm)"
  Limiting Max Torque/1 -> Gain3/1, Switch2/1, Mux/2, Product/1, Switch1/2  "T (Nm)"
  Gain1/1 -> Mux/1  "P (kW)"
  Mux/1 -> Parameters/1
  Gain3/1 -> Abs/1
  Gain4/1 -> Abs1/1
  Abs/1 -> Mot_Efficiency/1(T_mot_norm)
  Abs1/1 -> Mot_Efficiency/2(w_mot_norm)
  Reciprocal/1 -> Switch1/1
  Constant/1 -> SOC Empty Check/3
  Switch2/1 -> SOC Empty Check/1
  SOC Empty Check/1 -> Two-Way Connection/1
  connections:
  Shaft/RConn1 -- Two-Way Connection/RConn1
  Power/RConn1 -- Two-Way Connection1/RConn1

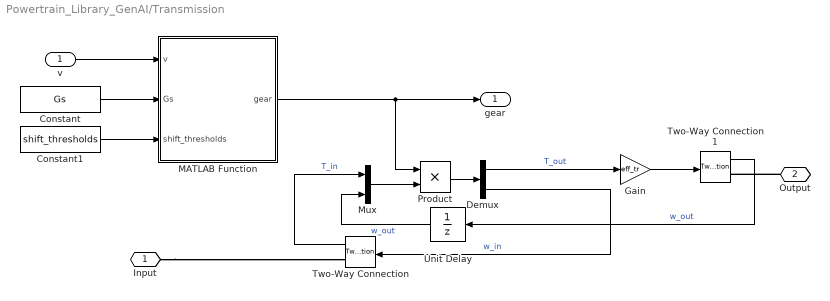
== system Powertrain_Library_GenAI/Transmission ==
  v : Inport
  Constant : Constant  Value=Gs
  Constant1 : Constant  Value=shift_thresholds
  Demux : Demux  Outputs=2
  Gain : Gain  Gain=eff_tr
  MATLAB Function : MATLAB Function  TreatAsAtomicUnit=on
  Mux : Mux  Inputs=2
  Product : Product
  Two-Way Connection : TwoWayConnection
  Two-Way Connection1 : TwoWayConnection
  Unit Delay : UnitDelay  SampleTime=-1  HasFrameUpgradeWarning=on
  Input : PMIOPort  Side=Left
  Output : PMIOPort  Port=2  Side=Right
  gear : Outport
  wires:
  Two-Way Connection/1 -> Mux/1  "T_in"
  Demux/1 -> Gain/1  "T_out"
  Mux/1 -> Product/2
  Product/1 -> Demux/1
  Demux/2 -> Two-Way Connection/1  "w_in"
  Two-Way Connection1/1 -> Unit Delay/1  "w_out"
  Constant/1 -> MATLAB Function/2(Gs)
  MATLAB Function/1(gear) -> gear/1, Product/1
  v/1 -> MATLAB Function/1(v)
  Constant1/1 -> MATLAB Function/3(shift_thresholds)
  Gain/1 -> Two-Way Connection1/1
  Unit Delay/1 -> Mux/2  "w_out"
  connections:
  Output/RConn1 -- Two-Way Connection1/RConn1
  Input/RConn1 -- Two-Way Connection/RConn1

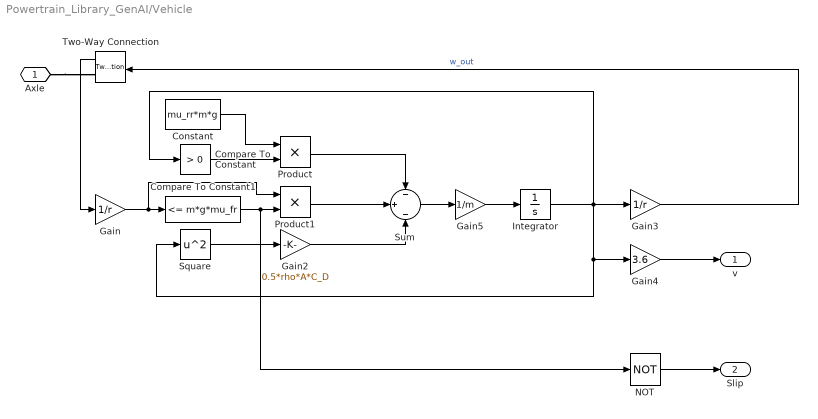
== system Powertrain_Library_GenAI/Vehicle ==
  Compare To Constant : simulink/Logic and Bit Operations/Compare To Constant  relop=>  const=0  OutDataTypeStr=uint8  ZeroCross=off
  Compare To Constant1 : simulink/Logic and Bit Operations/Compare To Constant  relop=<=  const=m*g*mu_fr  OutDataTypeStr=uint8  ZeroCross=off
  Constant : Constant  Value=mu_rr*m*g
  Gain : Gain  Gain=1/r
  Gain2 : Gain  Gain=0.5*rho*A*C_D
  Gain3 : Gain  Gain=1/r
  Gain4 : Gain  Gain=3.6
  Gain5 : Gain  Gain=1/m
  Integrator : Integrator
  NOT : Logic  Operator=NOT  IconShape=distinctive  AllPortsSameDT=off  OutDataTypeStr=boolean
  Product : Product
  Product1 : Product
  Square : Math  Operator=square
  Sum : Sum  Inputs=-|+|-
  Two-Way Connection : TwoWayConnection
  Axle : PMIOPort  Side=Left
  v : Outport
  Slip : Outport  Port=2
  wires:
  Gain2/1 -> Sum/3
  Gain/1 -> Product1/1, Compare To Constant1/1
  Compare To Constant/1 -> Product/2
  Gain5/1 -> Integrator/1
  Square/1 -> Gain2/1
  Sum/1 -> Gain5/1
  Gain4/1 -> v/1
  Integrator/1 -> Square/1, Gain4/1, Compare To Constant/1, Gain3/1
  Product/1 -> Sum/1
  Constant/1 -> Product/1
  Compare To Constant1/1 -> NOT/1, Product1/2
  Product1/1 -> Sum/2
  NOT/1 -> Slip/1
  Gain3/1 -> Two-Way Connection/1  "w_out"
  Two-Way Connection/1 -> Gain/1
  connections:
  Axle/RConn1 -- Two-Way Connection/RConn1

== system Powertrain_Library_GenAI/IC Engine/ICE_Efficiency ==
  T_ice_norm : Inport
  w_ice_pnorm : Inport  Port=2
  Average Efficiency : Subsystem  VariantControl=Constant Efficiency
  Efficiency Map : Subsystem  VariantControl=Variable Efficiency
  eff_ice : Outport
